simulink model "smdsim"  (R2016a)
settings: Solver=FixedStepDiscrete  StartTime=0.0  StopTime=10.0  FixedStep=0.1  RelTol=1e-3
settings Model: Creator=Samvrit  LastModifiedBy=Rohan computers
settings SolverCC: AutoInsertRateTranBlk=on
settings DataIOCC: LimitDataPoints=on
settings DebuggingCC: AllowSymbolicDim=off
settings ConfigComp: CovModelRefEnable=Off  CovSFcnEnable=off

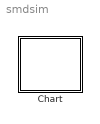
== system smdsim ==
  Chart : Stateflow chart  TreatAsAtomicUnit=on

== stateflow chart smdsim/Chart ==
  state IDLE
  state RETRIEVE_JOINT_VELOCITIES
  state SAVE_SIMULINK_FILE
  state RETRIEVE_JOINT_ANGLES
  state MODIFY_BLOCK_PARAMETERS
  state OPEN_SIMULINK_FILE
  state RUN_SIMULATION
  (default) -> IDLE
  SAVE_SIMULINK_FILE -> IDLE
  IDLE -> RETRIEVE_JOINT_ANGLES : simulate_button_press
  RETRIEVE_JOINT_ANGLES -> RETRIEVE_JOINT_VELOCITIES
  RUN_SIMULATION -> SAVE_SIMULINK_FILE
  RETRIEVE_JOINT_VELOCITIES -> OPEN_SIMULINK_FILE
  OPEN_SIMULINK_FILE -> MODIFY_BLOCK_PARAMETERS
  MODIFY_BLOCK_PARAMETERS -> RUN_SIMULATION
